simulink model "USV"  (R2022a)
settings: Solver=ode4  StartTime=0.0  StopTime=inf  FixedStep=0.001  RelTol=1e-3
PreLoadFcn:
  | [filepath,name,ext]  = fileparts(get_param(bdroot, 'FileName'));
  | InitFileName=[name,'_init.m'];
  | cd(filepath);
InitFcn:
  | [filepath,name,ext]  = fileparts(get_param(bdroot, 'FileName'));
  | InitFileName=[name,'_init.m'];
  | cd(filepath);
  | try
  | run(InitFileName);
  | end
values from neighbouring files (symbols this model uses):
  BoatParam_cf = 0.1    [USV_init.m]
  BoatParam_cg = 0.1    [USV_init.m]
  BoatParam_len = 1.5    [USV_init.m]
  BoatParam_lenSlope = pi/6    (= 0.523598775598)    [USV_init.m]
  BoatParam_waterDensity = 1000    [USV_init.m]
  BoatParam_widSlope = pi/4    (= 0.785398163397)    [USV_init.m]
  BoatParam_width = 0.8    [USV_init.m]
  ModelPara_coborigin = [0;0;0]    [USV_init.m]
  ModelParam_envAltitude = -600    [USV_init.m]
  ModelParam_GPSEphFinal = 0.3    [USV_init.m]
  ModelParam_GPSEpvFinal = 0.4    [USV_init.m]
  ModelParam_noiseGPSSampTime = 0.2    [USV_init.m]
  ModelParam_noisePowerOffGainAccel = 0.04    [USV_init.m]
  ModelParam_noisePowerOffGainAccelZ = 0.03    [USV_init.m]
  ModelParam_noisePowerOffGainGyro = 0.02    [USV_init.m]
  ModelParam_noisePowerOffGainGyroZ = 0.025    [USV_init.m]
  ModelParam_noisePowerOffGainMag = 0.02    [USV_init.m]
  ModelParam_noisePowerOffGainMagZ = 0.035    [USV_init.m]
  ModelParam_noisePowerOnGainAccel = 0.8    [USV_init.m]
  ModelParam_noisePowerOnGainAccelZ = 4.5    [USV_init.m]
  ModelParam_noisePowerOnGainGyro = 2    [USV_init.m]
  ModelParam_noisePowerOnGainGyroZ = 1    [USV_init.m]
  ModelParam_noisePowerOnGainMag = 0.025    [USV_init.m]
  ModelParam_noisePowerOnGainMagZ = 0.05    [USV_init.m]
  ModelParam_noiseUpperGPS = 0.5    [USV_init.m]
  ModelParam_uavCCm = [1 1 1]*200    [USV_init.m]
  ModelParam_uavCd = [2 200 200]    [USV_init.m]
  ModelParam_uavDearo = -0    (= 0)    [USV_init.m]
  ModelParam_uavMass = 227    [USV_init.m]
  ModelParam_uavType = int16(608)    [USV_init.m]
  motor = [motor,motorTmp]    [USV_init.m]
undefined symbols (not defined in the file or in its folder): Earth, ModelParam_GPSEpvInitial, ModelParam_GPSEpvTimeConstant, ModelParam_timeSamp, Newton, Raphson, USVPara, WGS84
libraries: RflySimModelLab x8, FaultUSVModelLib x4, aerolibtransform2 x4, vrlib x4, sharedutil x3, aerolibasang x3, sharedtransform x2, shared6dof x1, aerolibatmos2 x1, aerolibconvert2 x1, aerolibobsolete x1, simulink x1
(part 2 of 2)

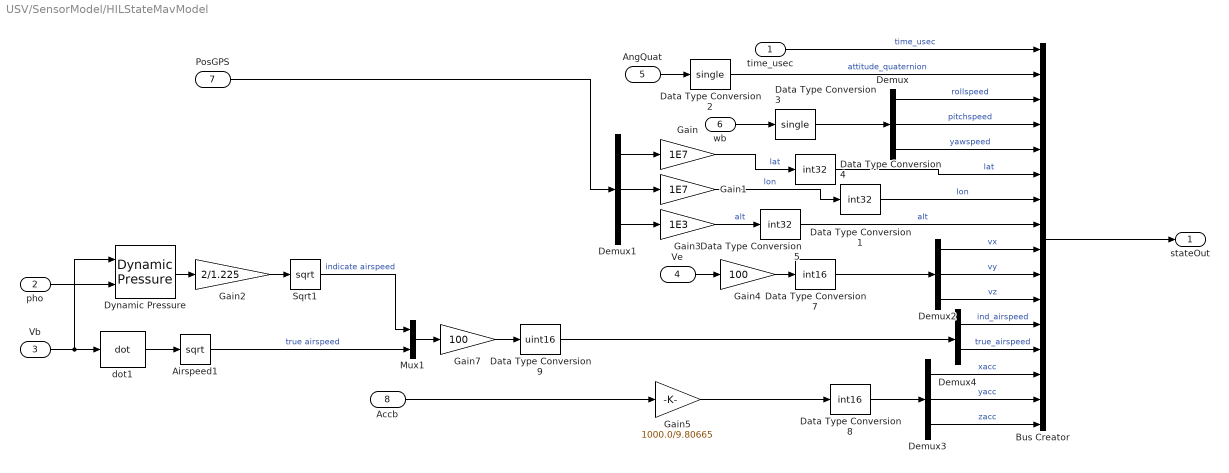
== system USV/SensorModel/HILStateMavModel ==
  time_usec : Inport
  pho : Inport  Port=2
  Vb : Inport  Port=3
  Ve : Inport  Port=4
  AngQuat : Inport  Port=5
  wb : Inport  Port=6
  PosGPS : Inport  Port=7
  Accb : Inport  Port=8
  Airspeed1 : Sqrt  AlgorithmType=Newton-Raphson
  Bus Creator : BusCreator  Inputs=16  OutDataTypeStr=Bus: MavLinkStateQuat  NonVirtualBus=on
  Data Type Conversion1 : DataTypeConversion  OutDataTypeStr=int32  RndMeth=Round  SaturateOnIntegerOverflow=off
  Data Type Conversion2 : DataTypeConversion  OutDataTypeStr=single  SaturateOnIntegerOverflow=off  RndMeth=Floor
  Data Type Conversion3 : DataTypeConversion  OutDataTypeStr=single  SaturateOnIntegerOverflow=off  RndMeth=Floor
  Data Type Conversion4 : DataTypeConversion  OutDataTypeStr=int32  RndMeth=Round  SaturateOnIntegerOverflow=off
  Data Type Conversion5 : DataTypeConversion  OutDataTypeStr=int32  RndMeth=Round  SaturateOnIntegerOverflow=off
  Data Type Conversion7 : DataTypeConversion  OutDataTypeStr=int16  RndMeth=Round  SaturateOnIntegerOverflow=off
  Data Type Conversion8 : DataTypeConversion  OutDataTypeStr=int16  RndMeth=Round  SaturateOnIntegerOverflow=off
  Data Type Conversion9 : DataTypeConversion  OutDataTypeStr=uint16  RndMeth=Round  SaturateOnIntegerOverflow=off
  Demux{,1..3} (4 alike) : Demux  Outputs=3
  Demux4 : Demux  Outputs=2
  Dynamic Pressure : aerolibasang/Dynamic Pressure
  Gain : Gain  Gain=1E7
  Gain1 : Gain  Gain=1E7
  Gain2 : Gain  Gain=2/1.225
  Gain3 : Gain  Gain=1E3
  Gain4 : Gain  Gain=100
  Gain5 : Gain  Gain=1000.0/9.80665
  Gain7 : Gain  Gain=100
  Mux1 : Mux  Inputs=2
  Sqrt1 : Sqrt
  dot1 : aerolibasang/Incidence, Sideslip, & Airspeed/dot  SystemSampleTime=-1  VariantActivationTime=update diagram  Latency=0  AutoFrameSizeCalculation=off
      settings: SourceProductBaseCode=AE
  stateOut : Outport  VectorParamsAs1DForOutWhenUnconnected=off
  wires:
  Sqrt1/1 -> Mux1/1  "indicate airspeed"
  Gain2/1 -> Sqrt1/1
  Dynamic Pressure/1 -> Gain2/1
  time_usec/1 -> Bus Creator/1  "time_usec"
  Vb/1 -> dot1/1, Dynamic Pressure/1
  AngQuat/1 -> Data Type Conversion2/1
  Ve/1 -> Gain4/1
  wb/1 -> Data Type Conversion3/1
  Airspeed1/1 -> Mux1/2  "true airspeed"
  Mux1/1 -> Gain7/1
  Demux4/1 -> Bus Creator/12  "ind_airspeed"
  Demux4/2 -> Bus Creator/13  "true_airspeed"
  Demux3/3 -> Bus Creator/16  "zacc"
  Demux3/2 -> Bus Creator/15  "yacc"
  Demux3/1 -> Bus Creator/14  "xacc"
  Gain5/1 -> Data Type Conversion8/1
  Accb/1 -> Gain5/1
  Demux2/3 -> Bus Creator/11  "vz"
  Demux2/2 -> Bus Creator/10  "vy"
  Demux2/1 -> Bus Creator/9  "vx"
  Gain4/1 -> Data Type Conversion7/1
  Gain3/1 -> Data Type Conversion5/1  "alt"
  Gain1/1 -> Data Type Conversion1/1  "lon"
  Gain/1 -> Data Type Conversion4/1  "lat"
  Demux1/3 -> Gain3/1
  Demux1/2 -> Gain1/1
  Demux1/1 -> Gain/1
  Demux/3 -> Bus Creator/5  "yawspeed"
  Demux/2 -> Bus Creator/4  "pitchspeed"
  Demux/1 -> Bus Creator/3  "rollspeed"
  Data Type Conversion2/1 -> Bus Creator/2  "attitude_quaternion"
  pho/1 -> Dynamic Pressure/2
  Gain7/1 -> Data Type Conversion9/1
  dot1/1 -> Airspeed1/1
  Data Type Conversion3/1 -> Demux/1
  Data Type Conversion7/1 -> Demux2/1
  Data Type Conversion9/1 -> Demux4/1
  Data Type Conversion8/1 -> Demux3/1
  Data Type Conversion4/1 -> Bus Creator/6  "lat"
  Data Type Conversion1/1 -> Bus Creator/7  "lon"
  Data Type Conversion5/1 -> Bus Creator/8  "alt"
  Bus Creator/1 -> stateOut/1
  PosGPS/1 -> Demux1/1

== system USV/Force and Moment Model/buoyancyModel/AirDrag ==
  <Vb> : Inport
  <wb> : Inport  Port=2
  Cp2MassDist : Inport  Port=3
  Body AeroCenter : MATLAB Function  TreatAsAtomicUnit=on
  ModelParam.uavCCm : Constant  Value=ModelParam_uavCCm
  ModelParam.uavCd : Constant  Value=ModelParam_uavCd
  Fb : Outport  VectorParamsAs1DForOutWhenUnconnected=off
  Mb : Outport  Port=2  VectorParamsAs1DForOutWhenUnconnected=off
  wires:
  Body AeroCenter/2(Md) -> Mb/1
  Body AeroCenter/1(Fd) -> Fb/1
  Cp2MassDist/1 -> Body AeroCenter/5(uavDearo)
  <wb>/1 -> Body AeroCenter/1(wb)
  <Vb>/1 -> Body AeroCenter/2(Vb)
  ModelParam.uavCd/1 -> Body AeroCenter/3(Cd)
  ModelParam.uavCCm/1 -> Body AeroCenter/4(CCm)

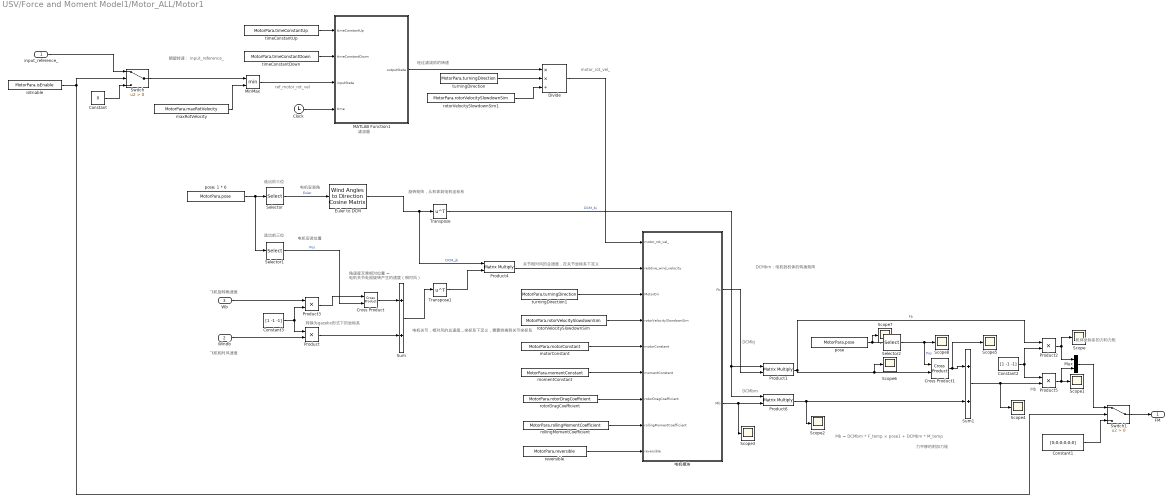
== system USV/Force and Moment Model1/Motor_ALL/Motor1 ==
  note: 选出前三位
  note: 期望转速：
      | input_reference_
  note: 滤波器
  note: 经过滤波后的转速
  note: ref_motor_rot_vel
  note: DCMbj
  note: Mb = DCMbm * F_temp × pose1 + DCMbm * M_temp
  note: DCMbm：电机到机体的转换矩阵
  note: DCMbm
  note: Mb
  note: 力平移的附加力矩
  note: 机体坐标系的力和力矩
  note: 转换为gazebo形式下的坐标系
  note: motor_rot_vel_
  note: 选出后三位
  note: 旋转矩阵，从机体到电机坐标系
  note: 电机安装角
  note: 电机安装位置
  note: 飞机相对风速度
  note: 飞机旋转角速度
  note: 角速度叉乘相对位置 = 电机关节处因旋转产生的速度（相对风）
  note: 电机关节，相对风的总速度，在机体坐标系下定义，需要转换到关节坐标系
  note: 关节相对风的总速度，在关节坐标系下定义
  input_reference_ : Inport
  Windb : Inport  Port=2
  Wb : Inport  Port=3
  Clock : Clock
  Constant : Constant  Value=0
  Constant1 : Constant  Value=[0;0;0;0;0;0]
  Constant2 : Constant  Value=[1 -1 -1]
  Constant3 : Constant  Value=[1 -1 -1]
  Cross Product : vrlib/Utilities/Cross Product
  Cross Product1 : vrlib/Utilities/Cross Product
  Divide : Product  Inputs=**/
  Euler to DCM : aerolibtransform2/Wind Angles to  Direction Cosine Matrix
      settings: SourceProductBaseCode=AE
  MATLAB Function1 : MATLAB Function  TreatAsAtomicUnit=on
  MinMax : MinMax  Inputs=2
  Mux : Mux  Inputs=2
  Product{,2..3,5} (4 alike) : Product
  Product1 : Product  Multiplication=Matrix(*)
  Product4 : Product  Multiplication=Matrix(*)
  Product6 : Product  Multiplication=Matrix(*)
  Scope{,1..8} (9 alike) : Scope
  Selector : Selector  InputPortWidth=6  IndexOptions=Starting index (dialog)  Indices=[4]  OutputSizes=3
  Selector1 : Selector  InputPortWidth=6  IndexOptions=Starting index (dialog)  Indices=[1]  OutputSizes=3
  Selector2 : Selector  InputPortWidth=6  IndexOptions=Starting index (dialog)  Indices=[1]  OutputSizes=3
  Sum : Sum
  Sum1 : Sum
  Switch : Switch  Criteria=u2 > Threshold  SaturateOnIntegerOverflow=off  InputSameDT=off
  Switch1 : Switch  Criteria=u2 > Threshold  SaturateOnIntegerOverflow=off  InputSameDT=off
  Transpose : Math  Operator=transpose  SignedPower=on
  Transpose1 : Math  Operator=transpose  SignedPower=on
  isEnable : Constant  Value=MotorPara.isEnable
  maxRotVelocity : Constant  Value=MotorPara.maxRotVelocity
  momentConstant : Constant  Value=MotorPara.momentConstant
  motorConstant : Constant  Value=MotorPara.motorConstant
  pose : Constant  Value=MotorPara.pose
  pose: 1 * 6 : Constant  Value=MotorPara.pose
  reversible : Constant  Value=MotorPara.reversible
  rollingMomentCoefficient : Constant  Value=MotorPara.rollingMomentCoefficient
  rotorDragCoefficient : Constant  Value=MotorPara.rotorDragCoefficient
  rotorVelocitySlowdownSim : Constant  Value=MotorPara.rotorVelocitySlowdownSim
  rotorVelocitySlowdownSim1 : Constant  Value=MotorPara.rotorVelocitySlowdownSim
  timeConstantDown : Constant  Value=MotorPara.timeConstantDown
  timeConstantUp : Constant  Value=MotorPara.timeConstantUp
  turningDirection : Constant  Value=MotorPara.turningDirection
  turningDirection1 : Constant  Value=MotorPara.turningDirection
  电机模块 : MATLAB Function  TreatAsAtomicUnit=on
  FM : Outport
  wires:
  Windb/1 -> Product/2
  Transpose/1 -> Product1/1, Product6/1  "DCM_bj"
  Switch1/1 -> FM/1
  Constant1/1 -> Switch1/3
  input_reference_/1 -> Switch/1
  Constant/1 -> Switch/3
  isEnable/1 -> Switch1/2, Switch/2
  Divide/1 -> 电机模块/1(motor_rot_vel_)
  reversible/1 -> 电机模块/9(reversible)
  Selector2/1 -> Scope8/1, Cross Product1/1  "Pos"
  pose/1 -> Scope7/1, Selector2/1
  Selector1/1 -> Cross Product/2  "Pos"
  Selector/1 -> Euler to DCM/1  "Euler"
  pose: 1 * 6/1 -> Selector/1, Selector1/1
  turningDirection/1 -> Divide/2
  rotorVelocitySlowdownSim1/1 -> Divide/3
  MATLAB Function1/1(outputState) -> Divide/1
  MinMax/1 -> MATLAB Function1/3(inputState)
  maxRotVelocity/1 -> MinMax/2
  Switch/1 -> MinMax/1
  Clock/1 -> MATLAB Function1/4(time)
  timeConstantUp/1 -> MATLAB Function1/1(timeConstantUp)
  timeConstantDown/1 -> MATLAB Function1/2(timeConstantDown)
  Transpose1/1 -> Product4/2
  Mux/1 -> Switch1/1
  Product6/1 -> Scope2/1, Sum1/2
  电机模块/2(Mb) -> Scope3/1, Product6/2
  Sum1/1 -> Scope4/1, Product5/2
  Cross Product1/1 -> Scope5/1, Sum1/1
  Product1/1 -> Product2/1, Scope6/1, Cross Product1/2  "Fb"
  电机模块/1(Fb) -> Product1/2
  Sum/1 -> Transpose1/1
  Product/1 -> Sum/2
  Cross Product/1 -> Sum/1
  Product3/1 -> Cross Product/1
  Wb/1 -> Product3/1
  Constant3/1 -> Product/1, Product3/2
  Euler to DCM/1 -> Transpose/1, Product4/1  "DCM_jb"
  Constant2/1 -> Product2/2, Product5/1
  Product5/1 -> Scope1/1, Mux/2
  Product2/1 -> Scope/1, Mux/1
  Product4/1 -> 电机模块/2(relative_wind_velocity)
  turningDirection1/1 -> 电机模块/3(MotorDir)
  rotorDragCoefficient/1 -> 电机模块/7(rotorDragCoefficient)
  momentConstant/1 -> 电机模块/6(momentConstant)
  motorConstant/1 -> 电机模块/5(motorConstant)
  rollingMomentCoefficient/1 -> 电机模块/8(rollingMomentCoefficient)
  rotorVelocitySlowdownSim/1 -> 电机模块/4(rotorVelocitySlowdownSim)

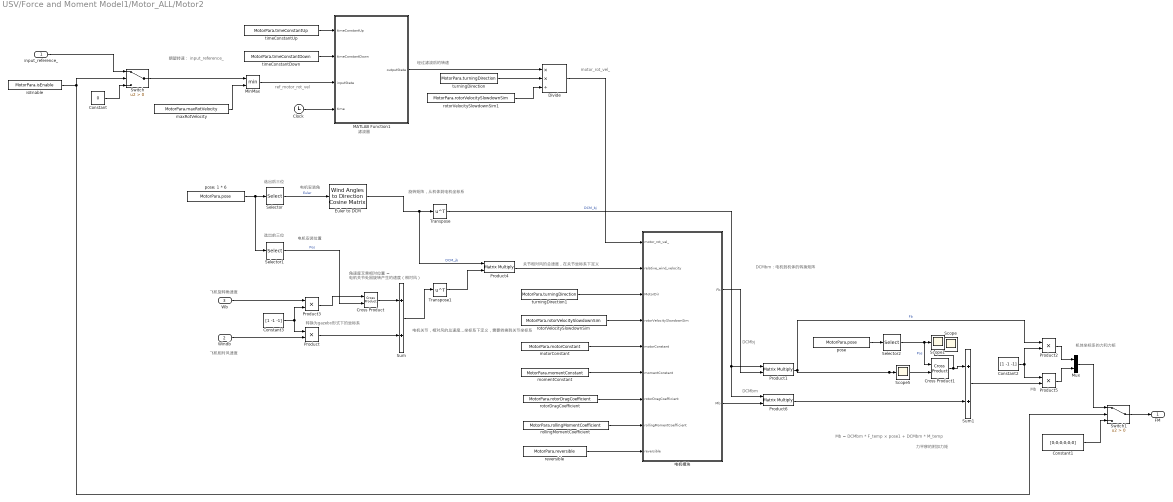
== system USV/Force and Moment Model1/Motor_ALL/Motor2 ==
  note: 选出前三位
  note: 期望转速：
      | input_reference_
  note: 滤波器
  note: 经过滤波后的转速
  note: ref_motor_rot_vel
  note: DCMbj
  note: Mb = DCMbm * F_temp × pose1 + DCMbm * M_temp
  note: DCMbm：电机到机体的转换矩阵
  note: DCMbm
  note: Mb
  note: 力平移的附加力矩
  note: 机体坐标系的力和力矩
  note: 转换为gazebo形式下的坐标系
  note: motor_rot_vel_
  note: 选出后三位
  note: 旋转矩阵，从机体到电机坐标系
  note: 电机安装角
  note: 电机安装位置
  note: 飞机相对风速度
  note: 飞机旋转角速度
  note: 角速度叉乘相对位置 = 电机关节处因旋转产生的速度（相对风）
  note: 电机关节，相对风的总速度，在机体坐标系下定义，需要转换到关节坐标系
  note: 关节相对风的总速度，在关节坐标系下定义
  input_reference_ : Inport
  Windb : Inport  Port=2
  Wb : Inport  Port=3
  Clock : Clock
  Constant : Constant  Value=0
  Constant1 : Constant  Value=[0;0;0;0;0;0]
  Constant2 : Constant  Value=[1 -1 -1]
  Constant3 : Constant  Value=[1 -1 -1]
  Cross Product : vrlib/Utilities/Cross Product
  Cross Product1 : vrlib/Utilities/Cross Product
  Divide : Product  Inputs=**/
  Euler to DCM : aerolibtransform2/Wind Angles to  Direction Cosine Matrix
      settings: SourceProductBaseCode=AE
  MATLAB Function1 : MATLAB Function  TreatAsAtomicUnit=on
  MinMax : MinMax  Inputs=2
  Mux : Mux  Inputs=2
  Product{,2..3,5} (4 alike) : Product
  Product1 : Product  Multiplication=Matrix(*)
  Product4 : Product  Multiplication=Matrix(*)
  Product6 : Product  Multiplication=Matrix(*)
  Scope : Scope
  Scope1 : Scope
  Scope5 : Scope
  Selector : Selector  InputPortWidth=6  IndexOptions=Starting index (dialog)  Indices=[4]  OutputSizes=3
  Selector1 : Selector  InputPortWidth=6  IndexOptions=Starting index (dialog)  Indices=[1]  OutputSizes=3
  Selector2 : Selector  InputPortWidth=6  IndexOptions=Starting index (dialog)  Indices=[1]  OutputSizes=3
  Sum : Sum
  Sum1 : Sum
  Switch : Switch  Criteria=u2 > Threshold  SaturateOnIntegerOverflow=off  InputSameDT=off
  Switch1 : Switch  Criteria=u2 > Threshold  SaturateOnIntegerOverflow=off  InputSameDT=off
  Transpose : Math  Operator=transpose  SignedPower=on
  Transpose1 : Math  Operator=transpose  SignedPower=on
  isEnable : Constant  Value=MotorPara.isEnable
  maxRotVelocity : Constant  Value=MotorPara.maxRotVelocity
  momentConstant : Constant  Value=MotorPara.momentConstant
  motorConstant : Constant  Value=MotorPara.motorConstant
  pose : Constant  Value=MotorPara.pose
  pose: 1 * 6 : Constant  Value=MotorPara.pose
  reversible : Constant  Value=MotorPara.reversible
  rollingMomentCoefficient : Constant  Value=MotorPara.rollingMomentCoefficient
  rotorDragCoefficient : Constant  Value=MotorPara.rotorDragCoefficient
  rotorVelocitySlowdownSim : Constant  Value=MotorPara.rotorVelocitySlowdownSim
  rotorVelocitySlowdownSim1 : Constant  Value=MotorPara.rotorVelocitySlowdownSim
  timeConstantDown : Constant  Value=MotorPara.timeConstantDown
  timeConstantUp : Constant  Value=MotorPara.timeConstantUp
  turningDirection : Constant  Value=MotorPara.turningDirection
  turningDirection1 : Constant  Value=MotorPara.turningDirection
  电机模块 : MATLAB Function  TreatAsAtomicUnit=on
  FM : Outport
  wires:
  Windb/1 -> Product/2
  Transpose/1 -> Product1/1, Product6/1  "DCM_bj"
  Switch1/1 -> FM/1
  Constant1/1 -> Switch1/3
  input_reference_/1 -> Switch/1
  Constant/1 -> Switch/3
  isEnable/1 -> Switch1/2, Switch/2
  Divide/1 -> 电机模块/1(motor_rot_vel_)
  reversible/1 -> 电机模块/9(reversible)
  Selector2/1 -> Scope1/1, Cross Product1/1  "Pos"
  pose/1 -> Selector2/1
  Selector1/1 -> Cross Product/2  "Pos"
  Selector/1 -> Euler to DCM/1  "Euler"
  pose: 1 * 6/1 -> Selector/1, Selector1/1
  turningDirection/1 -> Divide/2
  rotorVelocitySlowdownSim1/1 -> Divide/3
  MATLAB Function1/1(outputState) -> Divide/1
  MinMax/1 -> MATLAB Function1/3(inputState)
  maxRotVelocity/1 -> MinMax/2
  Switch/1 -> MinMax/1
  Clock/1 -> MATLAB Function1/4(time)
  timeConstantUp/1 -> MATLAB Function1/1(timeConstantUp)
  timeConstantDown/1 -> MATLAB Function1/2(timeConstantDown)
  Transpose1/1 -> Product4/2
  Mux/1 -> Switch1/1
  Product6/1 -> Sum1/2
  电机模块/2(Mb) -> Product6/2
  Sum1/1 -> Product5/2
  Cross Product1/1 -> Scope/1, Sum1/1
  Product1/1 -> Product2/1, Scope5/1, Cross Product1/2  "Fb"
  电机模块/1(Fb) -> Product1/2
  Sum/1 -> Transpose1/1
  Product/1 -> Sum/2
  Cross Product/1 -> Sum/1
  Product3/1 -> Cross Product/1
  Wb/1 -> Product3/1
  Constant3/1 -> Product/1, Product3/2
  Euler to DCM/1 -> Transpose/1, Product4/1  "DCM_jb"
  Constant2/1 -> Product2/2, Product5/1
  Product5/1 -> Mux/2
  Product2/1 -> Mux/1
  Product4/1 -> 电机模块/2(relative_wind_velocity)
  turningDirection1/1 -> 电机模块/3(MotorDir)
  rotorDragCoefficient/1 -> 电机模块/7(rotorDragCoefficient)
  momentConstant/1 -> 电机模块/6(momentConstant)
  motorConstant/1 -> 电机模块/5(motorConstant)
  rollingMomentCoefficient/1 -> 电机模块/8(rollingMomentCoefficient)
  rotorVelocitySlowdownSim/1 -> 电机模块/4(rotorVelocitySlowdownSim)

== system USV/SensorModel/HILGPSModel/NoiseFilter1 ==
  In1 : Inport
  Demux : Demux  Outputs=3
  Mux1 : Mux  Inputs=3
  Transfer Fcn1 : TransferFcn  Denominator=[0.05 1]
  Transfer Fcn2 : TransferFcn  Denominator=[0.05 1]
  Transfer Fcn4 : TransferFcn  Denominator=[0.05 1]
  Out1 : Outport  VectorParamsAs1DForOutWhenUnconnected=off
  wires:
  Mux1/1 -> Out1/1
  In1/1 -> Demux/1
  Demux/3 -> Transfer Fcn2/1
  Transfer Fcn4/1 -> Mux1/1
  Transfer Fcn2/1 -> Mux1/3
  Demux/1 -> Transfer Fcn4/1
  Transfer Fcn1/1 -> Mux1/2
  Demux/2 -> Transfer Fcn1/1

== system USV/SensorModel/HILGPSModel/NoiseFilter2 ==
  In1 : Inport
  Demux : Demux  Outputs=3
  Mux1 : Mux  Inputs=3
  Transfer Fcn1 : TransferFcn  Denominator=[0.05 1]
  Transfer Fcn2 : TransferFcn  Denominator=[0.05 1]
  Transfer Fcn4 : TransferFcn  Denominator=[0.05 1]
  Out1 : Outport  VectorParamsAs1DForOutWhenUnconnected=off
  wires:
  Mux1/1 -> Out1/1
  In1/1 -> Demux/1
  Demux/3 -> Transfer Fcn2/1
  Transfer Fcn4/1 -> Mux1/1
  Transfer Fcn2/1 -> Mux1/3
  Demux/1 -> Transfer Fcn4/1
  Transfer Fcn1/1 -> Mux1/2
  Demux/2 -> Transfer Fcn1/1

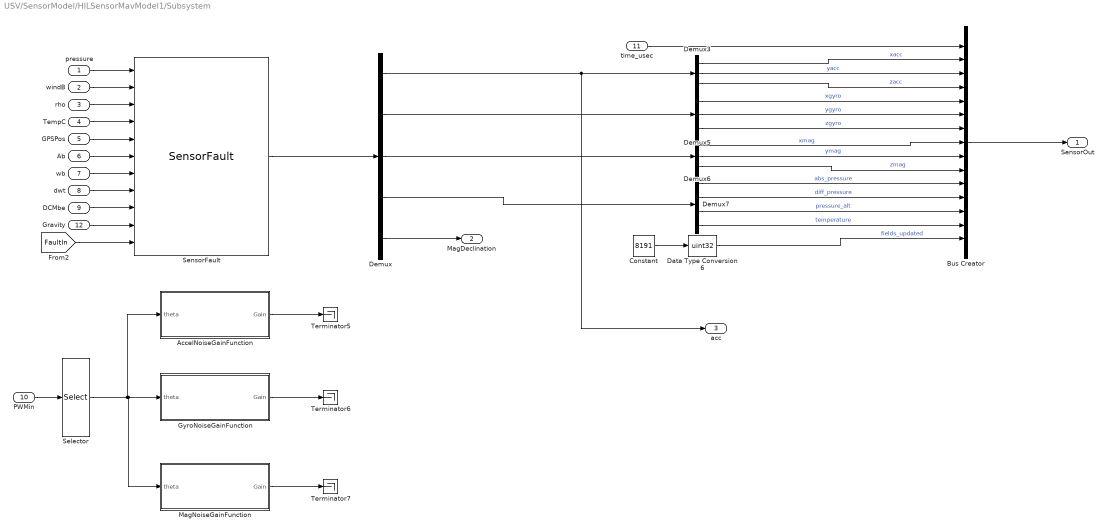
== system USV/SensorModel/HILSensorMavModel1/Subsystem ==
  pressure : Inport
  windB : Inport  Port=2
  rho : Inport  Port=3
  TempC : Inport  Port=4
  GPSPos : Inport  Port=5
  Ab : Inport  Port=6
  wb : Inport  Port=7
  dwt : Inport  Port=8
  DCMbe : Inport  Port=9
  PWMin : Inport  Port=10
  time_usec : Inport  Port=11
  Gravity : Inport  Port=12
  AccelNoiseGainFunction : MATLAB Function  TreatAsAtomicUnit=on
  Bus Creator : BusCreator  Inputs=15  OutDataTypeStr=Bus: MavLinkSensor  NonVirtualBus=on
  Constant : Constant  Value=8191
  Data Type Conversion6 : DataTypeConversion  OutDataTypeStr=uint32  SaturateOnIntegerOverflow=off  RndMeth=Floor
  Demux : Demux  Outputs=5
  Demux3 : Demux  Outputs=3
  Demux5 : Demux  Outputs=3
  Demux6 : Demux  Outputs=3
  Demux7 : Demux
  GyroNoiseGainFunction : MATLAB Function  TreatAsAtomicUnit=on
  MagNoiseGainFunction : MATLAB Function  TreatAsAtomicUnit=on
  Selector : Selector  InputPortWidth=8  IndexOptions=Index vector (dialog)  Indices=[1]  OutputSizes=1
  SensorFault : FaultUSVModelLib/SensorFault  FaultParamStruct=SensorFault  ComParamVect=FaultParamAPI
      link override Gain1: Gain=0.01
  Terminator5 : Terminator
  Terminator6 : Terminator
  Terminator7 : Terminator
  SensorOut : Outport  VectorParamsAs1DForOutWhenUnconnected=off
  MagDeclination : Outport  Port=2  VectorParamsAs1DForOutWhenUnconnected=off
  acc : Outport  Port=3  VectorParamsAs1DForOutWhenUnconnected=off
  wires:
  Selector/1 -> AccelNoiseGainFunction/1(theta), MagNoiseGainFunction/1(theta), GyroNoiseGainFunction/1(theta)
  AccelNoiseGainFunction/1(Gain) -> Terminator5/1
  Demux6/1 -> Bus Creator/8  "xmag"
  Demux6/3 -> Bus Creator/10  "zmag"
  Demux5/1 -> Bus Creator/5  "xgyro"
  Bus Creator/1 -> SensorOut/1
  Demux3/1 -> Bus Creator/2  "xacc"
  Demux7/3 -> Bus Creator/13  "pressure_alt"
  Demux5/3 -> Bus Creator/7  "zgyro"
  Demux7/2 -> Bus Creator/12  "diff_pressure"
  Demux3/3 -> Bus Creator/4  "zacc"
  wb/1 -> SensorFault/7
  Demux7/1 -> Bus Creator/11  "abs_pressure"
  Demux3/2 -> Bus Creator/3  "yacc"
  PWMin/1 -> Selector/1
  MagNoiseGainFunction/1(Gain) -> Terminator7/1
  Ab/1 -> SensorFault/6
  GyroNoiseGainFunction/1(Gain) -> Terminator6/1
  Demux7/4 -> Bus Creator/14  "temperature"
  Demux5/2 -> Bus Creator/6  "ygyro"
  TempC/1 -> SensorFault/4
  Demux6/2 -> Bus Creator/9  "ymag"
  Constant/1 -> Data Type Conversion6/1
  Data Type Conversion6/1 -> Bus Creator/15  "fields_updated"
  time_usec/1 -> Bus Creator/1
  pressure/1 -> SensorFault/1
  windB/1 -> SensorFault/2
  rho/1 -> SensorFault/3
  GPSPos/1 -> SensorFault/5
  dwt/1 -> SensorFault/8
  DCMbe/1 -> SensorFault/9
  Gravity/1 -> SensorFault/10
  [FaultIn] -> SensorFault/11
  SensorFault/1 -> Demux/1
  Demux/1 -> acc/1, Demux3/1
  Demux/2 -> Demux5/1
  Demux/3 -> Demux6/1
  Demux/4 -> Demux7/1
  Demux/5 -> MagDeclination/1

== matlab function USV/Force and Moment Model/buoyancyModel/MATLAB Function ==
  data: M input; fuPos output; wM output; rho input; cf input; dw input; alpha input; lw input; beta input; phi input; theta input; dz input
function [fuPos,wM] = fcn(M,rho,cf,dw,alpha,lw,beta,phi,theta,dz)
% M 船体的质量，重量的Mg
% rho 水的密度
% cf 船体当前浮心的位置，向下为正，北东地/前右下坐标系
% dw 船吃水处的宽度 d_water
% alpha 船吃水处的侧边沿与水面的夹角（船外边沿倾角）
% lw  船吃水处的长度 l_water
% beta 船吃水处的前后边沿与水面的夹角（船前边沿倾角）
% phi 船的滚转角，右手定则，向右滚（瞬时针）为正
% theta 船的俯仰角，右手定则
% dz 船身上下浮动的位移，向下为正

%% 进行输入角度限幅
% 将角度范围映射到-180 ~ 180 度
while phi>pi
    phi = phi -2*pi;
end
while phi<-pi
    phi = phi +2*pi;
end


% 将角度范围映射到-180 ~ 180 度
while theta>pi
    theta = theta -2*pi;
end
while theta<-pi
    theta = theta +2*pi;
end

% 滚转角限幅
if phi>pi/4 %如果大于45度，加上限幅
    phi=pi/4;
end

if phi<-pi/4 %如果小于-45度，加上限幅
    phi=-pi/4;
end

% 俯仰角限幅
if theta>pi/4 %如果大于45度，加上限幅
    theta=pi/4;
end

if theta<-pi/4  %如果小于-45度，加上限幅
    theta=-pi/4;
end


%% 计算左右翻转时，浮力的变化函数

% 浮心处的船等效长度
lw_e = lw-2*cf*cot(beta);


% 为避免浮心设置不合理导致，等效浮心失真，这里加入一个下限0.5倍
if lw_e < 0.5*lw
    lw_e = lw;
end


% 计算横截面和纵截面的等效面积
Std = M/(rho*lw_e);

% 看一下船是向左翻，还是向右翻
if phi<0 % 如果向左
    phi=abs(phi);
    roll_sign=1;
else %如果向右
    phi=abs(phi);
    roll_sign=-1;    
end

% 下面的推导是基于向左滚转的，在浮心输出时，需要做下映射

% 右侧排水减小面积和质心
dw_r = dw/2/(cos(phi)+sin(phi)*cot(alpha));
dw_r_e = (dw/2+dw_r)/2;

S_dr = dw_r_e*dw_r_e*sin(phi)/2;

y_dr = 2/3*dw_r_e*sin(phi/2);
z_dr =  2/3*dw_r_e*cos(phi/2);


% 左侧排水增加面积和质心
dw_l = dw/2*(cos(phi)+sin(phi)*cot(alpha-phi));
dw_l_e = (dw/2+dw_l)/2;

S_dl = dw_l_e*dw_l_e*sin(phi)/2;

y_dl = -2/3*dw_l_e*sin(phi/2);
z_dl =  -2/3*dw_l_e*cos(phi/2);

% 计算因左右侧排水面积（体积）差异，而产生的浮心变化

cf_z1 = (Std*cf - S_dr*z_dr + S_dl*z_dl)/Std;
cf_y = (-S_dr*y_dr + S_dl*y_dl)/Std;

% 左右倾斜情况下，浮心的位置所有区别
% 向左倾斜时，浮心应该左移，那么cf_y应该为负值
cf_y = cf_y*roll_sign;


%% 计算前后翻转时，浮力的变化函数
% 浮心处的船等效宽度
dw_e = dw-2*cf*cot(alpha);

if dw_e < 0.5*dw
    dw_e = dw;
end

Stl = M/(rho*dw_e);

% 看一下船是向前翻，还是向后翻
if theta<0 % 如果向前
    theta=abs(theta);
    pitch_sign=1;
else %如果向后
    theta=abs(theta);
    pitch_sign=-1;    
end

% 下面的推导是基于向前滚转的，在浮心输出时，需要做下映射

% 后侧排水减小面积和质心
lw_b = lw/2/(cos(theta)+sin(theta)*cot(beta));
lw_b_e = (lw/2+lw_b)/2;

S_db = lw_b_e*lw_b_e*sin(theta)/2;

y_db = 2/3*lw_b_e*sin(theta/2);
z_db =  2/3*lw_b_e*cos(theta/2);


% 前侧排水增加面积和质心
lw_f = lw/2*(cos(theta)+sin(theta)*cot(beta-theta));
lw_f_e = (lw/2+lw_f)/2;

S_df = lw_f_e*lw_f_e*sin(theta)/2;

y_df = -2/3*lw_f_e*sin(theta/2);
z_df =  -2/3*lw_f_e*cos(theta/2);

% 计算因前后侧排水面积（体积）差异，而产生的浮心变化

cf_z2 = (Stl*cf - S_db*z_db + S_df*z_df)/Stl;
cf_x = (-S_db*y_db + S_df*y_df)/Stl;

% 前后倾斜情况下，浮心的位置所有区别
% 向后倾斜时，浮心应该后移，那么cf_x应该为负值
cf_x = cf_x*pitch_sign;

% cf_z1
% cf_z2
%% 对浮心位置进行整合
fuPos=[cf_x,cf_y,cf_z1+cf_z2-cf];


%% 计算因船身倾转浮力质量的增加值
dM0 = (S_dl - S_dr)/Std*M; % 左右方向倾转，产生的额外排水质量
dM1 = (S_df - S_db)/Stl*M;% 左右方向倾转，产生的额外排水质量

% 假设船体为矩形，计算一个安全排水高度，作为阈值
h_max = Std/dw_e/lw_e; % 计算一个安全阈值，以此作为船的最底部

if dz > h_max % 认为船已经离开水面
    fuPos=[0,0,cf]; %浮心在默认位置
    wM=0; % 排水质量为0
    return;
end


% 假设船体为等腰梯形截面，底边为dw，底角为alpha，三角体的高度 = 船身等效长度lw_e
% 梯形的短边
dw1 = dw -dz*cot(alpha)*2;
%梯形面积公式
Sdz = dz*(dw+dw1)/2;
%梯形排水重心（浮心）公式
cf_dz = dz*(dw1+2*dw)/3/(dw1+dw);

cf_z2=(Std*cf-Sdz*cf_dz)/(Std-Sdz);

dM2 = -Sdz/Std*M;

wM=M+dM0+dM1+dM2;
if wM<0
    wM=0;
end
if wM >3*M %最大产生三倍重力
    wM = 3*wM;
end

fuPos(3)=fuPos(3)+(cf_z2-cf); % 加上浮心偏移量

== matlab function USV/SensorModel/HILGPSModel/GenCogVel ==
  data: v output; u input; cot output
function [v,cot] = Ang360(u)
v=norm(u(1:2));

if v < 1
    cot = 0;
else
    cot=atan2d(u(2),u(1));
end
 
if cot<0
    cot=cot+360;
end

== matlab function USV/SensorModel/HILGPSModel/MATLAB Function ==
  data: eph input; FixType output
function FixType = fcn(eph)
if eph <= 2
    FixType=3;
elseif eph <= 4
    FixType=2;
else
    FixType=0;
end

== matlab function USV/Force and Moment Model1/USV/FkAmassVec（根据USV） ==
  settings: updateMethod=DISCRETE
  data: Ma input; kAccelLinear input; F1 output; kAccelAngular input; M1 output
function [F1,M1] = fcn( Ma,kAccelLinear,kAccelAngular)

F1=[0;0;0];
M1=[0;0;0];

accV=[kAccelLinear(1);kAccelLinear(2);kAccelLinear(3);
    kAccelAngular(1);kAccelAngular(2);kAccelAngular(3)];
%线加速度和角加速度
%附加质量
FkAmassVec=-1.0 * Ma * accV;
F1=FkAmassVec(1:3);
M1=FkAmassVec(4:6);

== matlab function USV/SensorModel/HILSensorMavModel1/Subsystem/AccelNoiseGainFunction ==
  data: theta input; Gain output; ModelParam_noisePowerOnGainAccel parameter; ModelParam_noisePowerOffGainAccel parameter; ModelParam_noisePowerOnGainAccelZ parameter; ModelParam_noisePowerOffGainAccelZ parameter
function Gain = fcn(theta, ModelParam_noisePowerOnGainAccel, ModelParam_noisePowerOffGainAccel,ModelParam_noisePowerOnGainAccelZ, ModelParam_noisePowerOffGainAccelZ)
%#codegen
if theta>0.1
Gain = [ModelParam_noisePowerOnGainAccel;ModelParam_noisePowerOnGainAccel;ModelParam_noisePowerOnGainAccelZ];
else
    Gain = [ModelParam_noisePowerOffGainAccel;ModelParam_noisePowerOffGainAccel;ModelParam_noisePowerOffGainAccelZ];
end

== matlab function USV/SensorModel/HILSensorMavModel1/Subsystem/MagNoiseGainFunction ==
  data: theta input; Gain output; ModelParam_noisePowerOnGainMag parameter; ModelParam_noisePowerOffGainMag parameter; ModelParam_noisePowerOnGainMagZ parameter; ModelParam_noisePowerOffGainMagZ parameter
function Gain = fcn(theta, ModelParam_noisePowerOnGainMag, ModelParam_noisePowerOffGainMag, ModelParam_noisePowerOnGainMagZ, ModelParam_noisePowerOffGainMagZ)
%#codegen
if theta>0.1
    Gain = [ModelParam_noisePowerOnGainMag;ModelParam_noisePowerOnGainMag;ModelParam_noisePowerOnGainMagZ];
else
    Gain = [ModelParam_noisePowerOffGainMag;ModelParam_noisePowerOffGainMag;ModelParam_noisePowerOffGainMagZ];
end

== matlab function USV/Force and Moment Model/buoyancyModel/AirDrag/Body AeroCenter ==
  data: Fd output; Md output; wb input; Vb input; Cd input; CCm input; uavDearo input
function [Fd,Md] = fcn(wb,Vb,Cd, CCm, uavDearo)
% This is control effectiveness model, where Fb is the force produced by motors, Mb is
% the moment produced by motors, and Fd is the resistance produced by the air.
% The gyroscopic torque is not considered here.
% uavDearo 机身重心位置，向下为正

 Fd = -Cd*Vb.*abs(Vb);%
 
 Mfd=[Fd(2)*uavDearo;-Fd(1)*uavDearo;0];
 
Md=-CCm.*wb.*abs(wb);
Md=Mfd+Md;
%  CCm=4.72e-3;
%  Md=-CCm*wb.*abs(wb)*0.5;%0.3
%  Md= Mfd+Md;
 
end

== matlab function USV/Force and Moment Model/BoatWaterDrag/MATLAB Function ==
  data: beta input; M output; V input
function M = fcn(beta,V)

M=[0,0,0];

if V > 0.01
    M(3)= V*beta*5;
end

== matlab function USV/SensorModel/ZLimit ==
  data: zt input; xe input; Xee output
function Xee = fcn(zt,xe)
Xee=xe;
if Xee(3)>zt
    Xee(3)=zt;
end

== matlab function USV/Force and Moment Model1/USV/浮力（根据USV） ==
  settings: updateMethod=DISCRETE
  data: cob_origin input; mg input; q input; Xe input; HullRadius input; Fb output; Mb output; WaterLevel input; BoatLength input; BoatWidth input; LengthN input; Gravity input; WaterDensity input
 function [Fb, Mb] = fcn(cob_origin, mg, q, Xe, HullRadius, WaterLevel, BoatLength, BoatWidth, LengthN, Gravity, WaterDensity)
% This is a ground model that can provides reaction force and reaction torque
% persistent z0;
% if isempty(z0)
%      z0=0;
% end
Fb=[0;0;0];
Mb=[0;0;0];
bpnt=[0;0;0];
X=[0;0;0];
Xp=[0 0 0 Xe(1);0 0 0 Xe(2);0 0 0 Xe(3);0 0 0 0];
%四元数转换成旋转矩阵
x=q(1);
y=q(2);
z=q(3);
w=q(4);
a=1-2.*y.*y-2.*z.*z; b=2.*x.*y-2.*z.*w; c=2.*x.*z+2.*y.*w; d=2.*x.*y+2.*z.*w; e=1-2.*x.*x-2.*z.*z; f=2.*y.*z-2.*x.*w; g=2.*x.*z-2.*y.*w; h=2.*y.*z+2.*x.*w; i=1-2.*x.*x-2.*y.*y;
xf=[a b c 0;d e f 0;g h i 0;0 0 0 1];%旋转矩阵，体坐标系到世界坐标系
%% 计算浮力
%xformV由R和t组成
xformV=xf+Xp;
for i=0:1
    bpnt(2)=(i.*2.0-1.0).*BoatWidth/2.0;
    for j=1:LengthN
       bpnt(1)=((((j - 0.5) /LengthN) - 0.5).*BoatLength);
       bpntW = xformV \ [bpnt;1];%这里求逆
       kDdz = Xe(3) + bpntW(3);

       dz = X(3);
       DZ = (WaterLevel + dz) - kDdz;
       DZ = max(DZ,-HullRadius);
       DZ = min(DZ,HullRadius);
       DZ=-DZ;
       Z=[0;0;DZ];
       %浮力
       Fbb=(HullRadius.^2.*acos(complex(HullRadius-Z)./HullRadius)-(HullRadius-Z).*(sqrt(abs(2.*HullRadius.*Z-(Z).^2 )))).*(BoatLength)./(LengthN).*Gravity.*WaterDensity;
       F=bpnt+Fbb;
       Mb = real(cross(F,-cob_origin));    % 力的平移，计算力矩
       % Fb=-mg-F;
       Fb=real(HullRadius.^2.*acos(complex(HullRadius-Z)./HullRadius)-(HullRadius-Z).*(sqrt(abs(2.*HullRadius.*Z-(Z).^2 ))));
       
    end
end

== matlab function USV/Force and Moment Model1/USV/阻力（根据USV） ==
  settings: updateMethod=DISCRETE
  data: waterwb input; waterb input; Dmat input; Vb input; F1 output; wb input; M1 output
function [F1,M1] = fcn(waterwb,waterb,Dmat,Vb,wb)
% This is a ground model that can provides reaction force and reaction torque

F1=[0;0;0];
M1=[0;0;0];
V=[Vb(1)-waterb(1);Vb(2)-waterb(2);Vb(3)-waterb(3);wb(1)-waterwb(1);wb(2)-waterwb(2);wb(3)-waterwb(3)];%线速度和角速度

%水的阻力
FkDvec = -1.0 * Dmat * V;
F1=FkDvec(1:3);
M1=FkDvec(4:6);

== matlab function USV/SensorModel/HILSensorMavModel1/Subsystem/GyroNoiseGainFunction ==
  data: theta input; Gain output; ModelParam_noisePowerOnGainGyro parameter; ModelParam_noisePowerOffGainGyro parameter; ModelParam_noisePowerOnGainGyroZ parameter; ModelParam_noisePowerOffGainGyroZ parameter
function Gain = fcn(theta, ModelParam_noisePowerOnGainGyro, ModelParam_noisePowerOffGainGyro, ModelParam_noisePowerOnGainGyroZ, ModelParam_noisePowerOffGainGyroZ)
%#codegen
if theta>0.1
    Gain = [ModelParam_noisePowerOnGainGyro;ModelParam_noisePowerOnGainGyro;ModelParam_noisePowerOnGainGyroZ];
else
    Gain = [ModelParam_noisePowerOffGainGyro;ModelParam_noisePowerOffGainGyro;ModelParam_noisePowerOffGainGyroZ];
end

== matlab function USV/Force and Moment Model/BoatWaterDrag/Body AeroCenter ==
  data: Fd output; Md output; wb input; Vb input; Cd input; CCm input; Dmat input
function [Fd,Md] = fcn(wb,Vb,Cd, CCm, Dmat)
% This is control effectiveness model, where Fb is the force produced by motors, Mb is
% the moment produced by motors, and Fd is the resistance produced by the air.
% The gyroscopic torque is not considered here.
% uavDearo 机身重心位置，向下为正

 %Mfd=cross(uavDearo',Fd);
 %Mfd=[Fd(2)*uavDearo;-Fd(1)*uavDearo;0];
%Md=Mfd+Md;
%  CCm=4.72e-3;
%  Md=-CCm*wb.*abs(wb)*0.5;%0.3
%  Md= Mfd+Md;
 
% -----------------------------
% Fd = -Cd'.*Vb.*abs(Vb);
% Md=-CCm.*wb.*abs(wb);
% -----------------------------

Fd=[0;0;0];
Md=[0;0;0];
V=[Vb(1);Vb(2);Vb(3);wb(1);wb(2);wb(3)];%线速度和角速度

%水的阻力
FkDvec = -1.0 * Dmat * V;
Fd=FkDvec(1:3);
Md=FkDvec(4:6);

== matlab function USV/Force and Moment Model1/Motor_ALL/Motor1/MATLAB Function1 ==
  settings: updateMethod=DISCRETE
  data: timeConstantUp input; outputState output; timeConstantDown input; inputState input; time input
function outputState = fcn(timeConstantUp, timeConstantDown, inputState, time)
persistent previousState;
if isempty(previousState)
    previousState=0;
end

persistent lastTime;
if isempty(lastTime)
    lastTime=0;
end

samplingTime=time-lastTime;
if samplingTime<=0
    samplingTime=0.01;
end

if inputState > previousState
    alphaUp = exp(-samplingTime/timeConstantUp);
    outputState = alphaUp*previousState + (1-alphaUp)*inputState;
else
    alphaDown = exp(- samplingTime / timeConstantDown);
    outputState = alphaDown*previousState + (1-alphaDown)*inputState;
end

previousState=inputState;
lastTime=time;

== matlab function USV/Force and Moment Model1/Motor_ALL/Motor1/电机模块 ==
  data: motor_rot_vel_ input; relative_wind_velocity input; MotorDir input; rotorVelocitySlowdownSim input; motorConstant input; momentConstant input; rotorDragCoefficient input; Fb output; Mb output; rollingMomentCoefficient input; reversible input
function [Fb,Mb] = fcn(motor_rot_vel_,relative_wind_velocity,MotorDir,...
    rotorVelocitySlowdownSim,motorConstant,momentConstant,rotorDragCoefficient,...
   rollingMomentCoefficient,reversible)
% This is control effectiveness model, where Fb is the force produced by motors, Mb is
% the moment produced by motors, and Fd is the resistance produced by the air.
% The gyroscopic torque is not considered here.

% -1: anticlockwise, 1: clockwise 

Mb = [0;0;0];
Fb = [0;0;0];

propdir = MotorDir;
real_motor_velocity = motor_rot_vel_ * rotorVelocitySlowdownSim;

% 相对风速分量
velocity_perpendicular_to_rotor_axis = [relative_wind_velocity(1);relative_wind_velocity(2);0];
velocity_parallel_to_rotor_axis = [0;0;relative_wind_velocity(3)];
vel = abs(relative_wind_velocity(3));
scalar = 1 - vel/25.0;
if scalar<0
    scalar = 0;
elseif scalar>1
        scalar = 0;
end
% 推力 % Fm应用到模型上之前还需要根据与水流/风速的相对速度进行缩放，scale：0-1
force = real_motor_velocity * abs(real_motor_velocity) * motorConstant;
if reversible==0          % 表示电机不能有负推力
    force = abs(force);
end
Fm1 = [0;0;force * scalar];
%  旋翼的气动阻力
% relative_wind_velocity = body_velocity - wind_vel_;
% velocity_perpendicular_to_rotor_axis = relative_wind_velocity - (relative_wind_velocity.*(joint_axis)) .* joint_axis;
Fm2 = -abs(real_motor_velocity) * rotorDragCoefficient * velocity_perpendicular_to_rotor_axis;
Fb = Fm1 + Fm2;

% 用于偏航的空气阻力矩  Mt1     
Mt1 = [0;0;-propdir*force*momentConstant];    % gazebo中ccw对应1，而这里对应-1，所以propdir前没负号
% 滚动力矩Mt2
Mt2 = -abs(real_motor_velocity) * rollingMomentCoefficient * velocity_perpendicular_to_rotor_axis;
Mb = Mt1 + Mt2;

end

== matlab function USV/Force and Moment Model1/Motor_ALL/Motor2/MATLAB Function1 ==
  settings: updateMethod=DISCRETE
  data: timeConstantUp input; outputState output; timeConstantDown input; inputState input; time input
function outputState = fcn(timeConstantUp, timeConstantDown, inputState, time)
persistent previousState;
if isempty(previousState)
    previousState=0;
end

persistent lastTime;
if isempty(lastTime)
    lastTime=0;
end

samplingTime=time-lastTime;
if samplingTime<=0
    samplingTime=0.01;
end

if inputState > previousState
    alphaUp = exp(-samplingTime/timeConstantUp);
    outputState = alphaUp*previousState + (1-alphaUp)*inputState;
else
    alphaDown = exp(- samplingTime / timeConstantDown);
    outputState = alphaDown*previousState + (1-alphaDown)*inputState;
end

previousState=inputState;
lastTime=time;

== matlab function USV/Force and Moment Model1/Motor_ALL/Motor2/电机模块 ==
  data: motor_rot_vel_ input; relative_wind_velocity input; MotorDir input; rotorVelocitySlowdownSim input; motorConstant input; momentConstant input; rotorDragCoefficient input; Fb output; Mb output; rollingMomentCoefficient input; reversible input
function [Fb,Mb] = fcn(motor_rot_vel_,relative_wind_velocity,MotorDir,...
    rotorVelocitySlowdownSim,motorConstant,momentConstant,rotorDragCoefficient,...
   rollingMomentCoefficient,reversible)
% This is control effectiveness model, where Fb is the force produced by motors, Mb is
% the moment produced by motors, and Fd is the resistance produced by the air.
% The gyroscopic torque is not considered here.

% -1: anticlockwise, 1: clockwise 

Mb = [0;0;0];
Fb = [0;0;0];

propdir = MotorDir;
real_motor_velocity = motor_rot_vel_ * rotorVelocitySlowdownSim;

% 相对风速分量
velocity_perpendicular_to_rotor_axis = [relative_wind_velocity(1);relative_wind_velocity(2);0];
velocity_parallel_to_rotor_axis = [0;0;relative_wind_velocity(3)];
vel = abs(relative_wind_velocity(3));
scalar = 1 - vel/25.0;
if scalar<0
    scalar = 0;
elseif scalar>1
        scalar = 0;
end
% 推力 % Fm应用到模型上之前还需要根据与水流/风速的相对速度进行缩放，scale：0-1
force = real_motor_velocity * abs(real_motor_velocity) * motorConstant;
if reversible==0          % 表示电机不能有负推力
    force = abs(force);
end
Fm1 = [0;0;force * scalar];
%  旋翼的气动阻力
% relative_wind_velocity = body_velocity - wind_vel_;
% velocity_perpendicular_to_rotor_axis = relative_wind_velocity - (relative_wind_velocity.*(joint_axis)) .* joint_axis;
Fm2 = -abs(real_motor_velocity) * rotorDragCoefficient * velocity_perpendicular_to_rotor_axis;
Fb = Fm1 + Fm2;

% 用于偏航的空气阻力矩  Mt1     
Mt1 = [0;0;-propdir*force*momentConstant];    % gazebo中ccw对应1，而这里对应-1，所以propdir前没负号
% 滚动力矩Mt2
Mt2 = -abs(real_motor_velocity) * rollingMomentCoefficient * velocity_perpendicular_to_rotor_axis;
Mb = Mt1 + Mt2;

end

== matlab function USV/Force and Moment Model1/OnGroundFaceup ==
  data: EulerAng input; y output
function y = fcn(EulerAng)

targetRoll = 0;
% if cos(EulerAng(1))<0
%     targetRoll=pi;  
% end

targetPitch = 0;
% if cos(EulerAng(2))<0
%         targetPitch=pi;
% end
    
y = [targetRoll;targetPitch;EulerAng(3)];
